simulink model "AutonomousDriving"  (R2018a)
settings: Solver=FixedStepAuto  StartTime=0.0  StopTime=inf  FixedStep=0.1  RelTol=1e-3
values from neighbouring files (symbols this model uses):
  init =     [init.mat]
undefined symbols (not defined in the file or in its folder): gray, Rec, SDTV
libraries: vrlib x7, visiontextngfix x4, visiontransforms x4, visiongeotforms x3, visionanalysis x3, visionstatistics x3, visionconversions x1
settings Model: Creator=al.hermann  LastModifiedBy=al.hermann

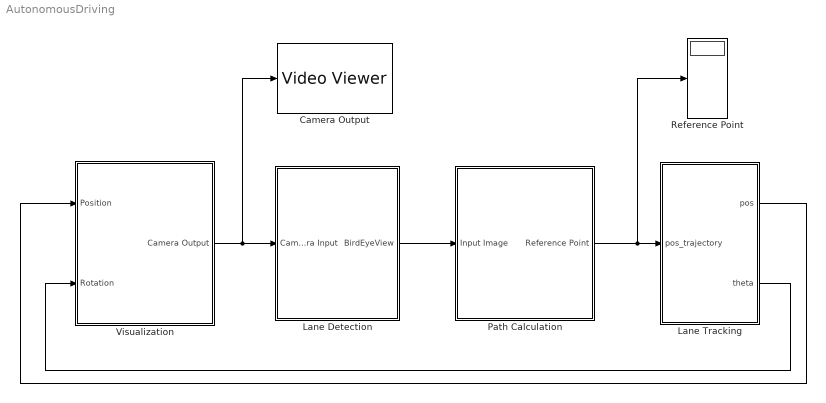
== system AutonomousDriving ==
  Camera Output : VideoViewer  colormapValue=gray(256)  FigPos=[1 481 575 361]
  Lane Detection : Subsystem
  Lane Tracking : Subsystem
  Path Calculation : Subsystem
  Reference Point : Display
  Visualization : Subsystem
  wires:
  Lane Detection/1(BirdEyeView) -> Path Calculation/1(Input Image)
  Lane Tracking/2(theta) -> Visualization/2(Rotation)
  Visualization/1(Camera Output) -> Lane Detection/1(Camera Input), Camera Output/1
  Lane Tracking/1(pos) -> Visualization/1(Position)
  Path Calculation/1("Reference Point ") -> Lane Tracking/1(pos_trajectory), Reference Point/1

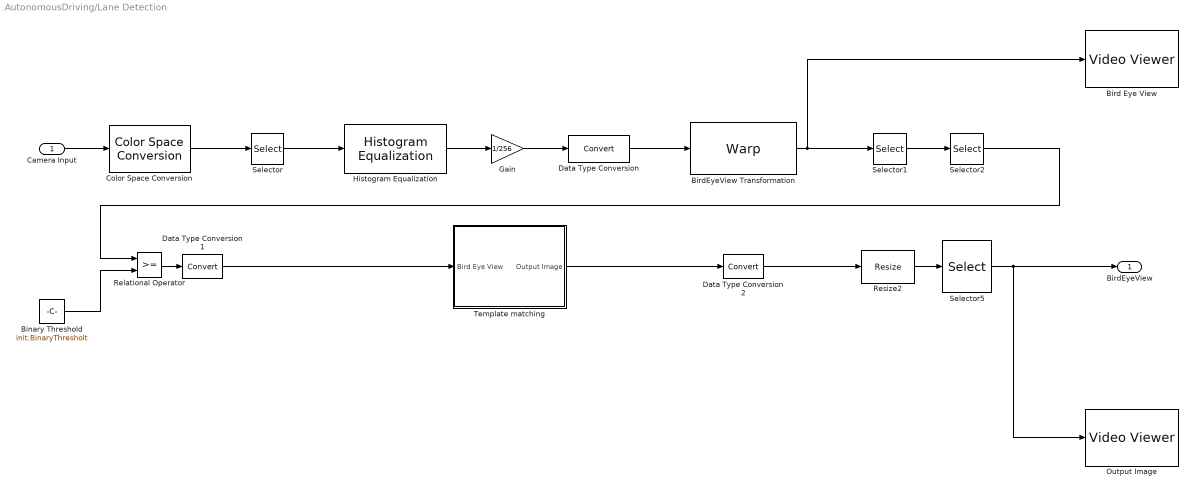
== system AutonomousDriving/Lane Detection ==
  Camera Input : Inport
  Binary Threshold : Constant  Value=init.BinaryThresholt
  Bird Eye View : VideoViewer  colormapValue=gray(256)  FigPos=[577 469 577 349]
  BirdEyeView Transformation : visiongeotforms/Warp  TransformMatrixSource=Custom  TransformMatrix=tf.T  InterpolationMethod=Bicubic  BackgroundFillValue=0  OutputImagePositionSource=Custom  OutputImagePosition=[-128, -128, 512, 512 ]  ROIInputPort=off  ROIValidityOutputPort=off  SimulateUsing=Interpreted execution
      settings: SourceProductName=Computer Vision System Toolbox  SourceProductBaseCode=VP
  Color Space Conversion : visionconversions/Color Space  Conversion  conversion=Obsolete  conversionActive=R'G'B' to intensity  wp_str=D65  rec=Rec. 601 (SDTV)  sys=1125/60/2:1  imagePorts=One multidimensional signal
      settings: SourceProductName=Computer Vision System Toolbox
  Data Type Conversion : DataTypeConversion
  Data Type Conversion1 : DataTypeConversion
  Data Type Conversion2 : DataTypeConversion
  Gain : Gain  Gain=1/256
  Histogram Equalization : visionanalysis/Histogram Equalization  specify=Uniform  numbins=256  src=Specify via dialog  hist=ones(1,64)
      settings: SourceProductName=Computer Vision System Toolbox  SourceProductBaseCode=VP
  Output Image : VideoViewer  colormapValue=gray(256)  FigPos=[519 965 488 384]
  Relational Operator : RelationalOperator  OutDataTypeStr=boolean  RndMeth=Simplest
  Resize2 : visiongeotforms/Resize  specify=Number of output rows and columns  rfactor=[500 100]  outCols=25  outRows=25  outRowsCols=init.ResizeImage  interp_method=Bilinear  antialias=on  useROI=off  roiFlag=off  prodOutputMode=Binary point scaling  prodOutputWordLength=32  prodOutputFracLength=10  roundingMode=Nearest  overflowMode=on
      settings: SourceProductName=Computer Vision System Toolbox  SourceProductBaseCode=VP
  Selector : Selector  NumberOfDimensions=2  InputPortWidth=3  IndexOptions=Starting index (dialog),Starting index (dialog)  Indices=100,50  OutputSizes=100,220
  Selector1 : Selector  NumberOfDimensions=2  InputPortWidth=3  IndexOptions=Starting index (dialog),Starting index (dialog)  Indices=244,1  OutputSizes=512-244,512
  Selector2 : Selector  NumberOfDimensions=2  InputPortWidth=3  IndexOptions=Starting index (dialog),Starting index (dialog)  Indices=1,1  OutputSizes=107,512
  Selector5 : Selector  NumberOfDimensions=2  InputPortWidth=3  IndexOptions=Starting index (dialog),Starting index (dialog)  Indices=25,50  OutputSizes=648-25,350
  Template matching : Subsystem
  BirdEyeView : Outport
  wires:
  Camera Input/1 -> Color Space Conversion/1
  Color Space Conversion/1 -> Selector/1
  Selector/1 -> Histogram Equalization/1
  Histogram Equalization/1 -> Gain/1
  Gain/1 -> Data Type Conversion/1
  Data Type Conversion/1 -> BirdEyeView Transformation/1
  Selector1/1 -> Selector2/1
  Relational Operator/1 -> Data Type Conversion1/1
  Binary Threshold/1 -> Relational Operator/2
  Data Type Conversion2/1 -> Resize2/1
  BirdEyeView Transformation/1 -> Selector1/1, Bird Eye View/1
  Selector2/1 -> Relational Operator/1
  Selector5/1 -> Output Image/1, BirdEyeView/1
  Resize2/1 -> Selector5/1
  Data Type Conversion1/1 -> Template matching/1(Bird Eye View)
  Template matching/1(Output Image) -> Data Type Conversion2/1

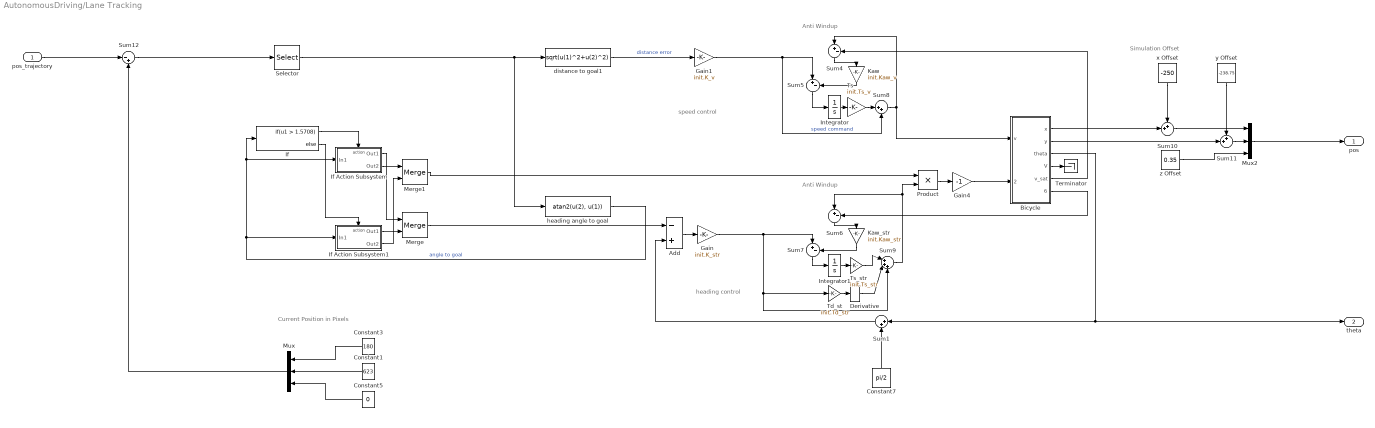
== system AutonomousDriving/Lane Tracking ==
  note: Simulation Offset
  note: Anti Windup
  note: Current Position in Pixels
  note: speed control
  note: heading control
  note: Anti Windup
  pos_trajectory : Inport
  Add : Sum  Inputs=-+
  Bicycle : Subsystem  AncestorBlock=roblocks/Vehicles/Bicycle  mask{vlim=init.v, accel=1, alim=120*pi/180, steer_rate=40*pi/180, L=2.812, x0=[0, 0, 0]}
      mask prompts: vlim "Velocity limit (m/s)"; accel "Acceleration limit (m/s2)"; alim "Steering angle limit (rad)"; steer_rate "Steering rate limit (rad/s)"; L "Wheel base"; x0 "Initial state (x, y, theta)"
      mask help: Kino-dynamic model of bicycle vehicle
      mask Help:
      | Kino-dynamic model of bicycle vehicle, also known as Ackermann vehicle
      | model.
      | 
      | <b>Parameters::</b>
      | 
      | Acceleration (1x1)   Vehicle acceleration limit [m/s2]
      | Velocity limit (1x1)  Vehicle speed limit [m/s]
      | Steering limits (1x1) Steering angle limit [rad]
      | Initial state (1x3) Initial state (x, y, theta)
      | Handbrake (1x1) Vehicle cannot move if non-zero
      | 
      | <b>Inputs::</b>
      | 
      | v (1x1) velocity demand [m/s]
      | gamma (1x1) steering angle [rad]
      | 
      | <b>Outputs::</b>
      | 
      | x (1x1) x-coordinate in world frame [m]
      | y (1x1) x-coordinate in world frame [m]
      | theta (1x1) heading angle in world frame [rad]
      | 
      | 
      | <b>Notes::</b>
      | 
      | - Steering limit is symmetric between -limit and +limit
      | - Same dynamic model as the Toolbox class Vehicle.
      mask Display:
      | port_label('input', 1, 'v')
      | port_label('input', 2, '\gamma', 'texmode', 'on')
      | port_label('output', 1, 'x')
      | port_label('output', 2, 'y')
      | port_label('output', 3, '\theta', 'texmode', 'on')
      | port_label('output', 4, 'v')
      | port_label('output', 5, 'v_{sat}', 'texmode', 'on')
      | port_label('output', 6, '\theta_{sat}', 'texmode', 'on')
  Constant1 : Constant  Value=623
  Constant3 : Constant  Value=180
  Constant5 : Constant  Value=0
  Constant7 : Constant  Value=pi/2
  Derivative : Derivative  CoefficientInTFapproximation=100
  Gain : Gain  Gain=init.K_str
  Gain1 : Gain  Gain=init.K_v
  Gain4 : Gain  Gain=-1
  If : If  IfExpression=u1 > 1.5708
  If Action Subsystem : Subsystem  TreatAsAtomicUnit=on
  If Action Subsystem1 : Subsystem  TreatAsAtomicUnit=on
  Integrator : Integrator
  Integrator1 : Integrator
  Kaw : Gain  Gain=init.Kaw_v
  Kaw_str : Gain  Gain=init.Kaw_str
  Merge : Merge
  Merge1 : Merge
  Mux : Mux  Inputs=3
  Mux2 : Mux  Inputs=3
  Product : Product
  Selector : Selector  InputPortWidth=3  IndexOptions=Index vector (dialog)  Indices=[1 2]  OutputSizes=1
  Sum1 : Sum  Inputs=|++
  Sum10 : Sum  Inputs=++|
  Sum11 : Sum  Inputs=++|
  Sum12 : Sum  Inputs=|-+
  Sum{4..7} (4 alike) : Sum  Inputs=|+-
  Sum8 : Sum  Inputs=|++
  Sum9 : Sum  Inputs=|+++
  Td_st : Gain  Gain=init.Td_str
  Terminator : Terminator
  Ts : Gain  Gain=init.Ts_v
  Ts_str : Gain  Gain=init.Ts_str
  distance to goal1 : Fcn  Expr=sqrt(u(1)^2+u(2)^2)
  heading angle to goal : Fcn  Expr=atan2(u(2), u(1))
  x Offset : Constant  Value=-250
  y Offset : Constant  Value=-238.75
  z Offset : Constant  Value=0.35
  pos : Outport
  theta : Outport  Port=2
  wires:
  pos_trajectory/1 -> Sum12/1
  distance to goal1/1 -> Gain1/1  "distance error"
  Bicycle/3(theta) -> Sum1/1, theta/1
  Sum12/1 -> Selector/1
  Selector/1 -> distance to goal1/1, heading angle to goal/1
  Mux/1 -> Sum12/2
  Constant1/1 -> Mux/2
  Constant3/1 -> Mux/1
  Constant7/1 -> Sum1/2
  Gain1/1 -> Sum8/2, Sum5/1  "speed command"
  Constant5/1 -> Mux/3
  Bicycle/1(x) -> Sum10/2
  Bicycle/2(y) -> Sum11/2
  If Action Subsystem/1(Out1) -> Merge/1
  If/1 -> If Action Subsystem/Action
  If/2 -> If Action Subsystem1/Action
  If Action Subsystem/2(Out2) -> Merge1/1
  If Action Subsystem1/1(Out1) -> Merge/2
  Bicycle/5("v_sat ") -> Sum4/2
  Sum4/1 -> Kaw/1
  Kaw/1 -> Sum5/2
  Sum5/1 -> Integrator/1
  Integrator/1 -> Ts/1
  Kaw_str/1 -> Sum7/2
  Sum7/1 -> Integrator1/1
  Sum6/1 -> Kaw_str/1
  Integrator1/1 -> Ts_str/1
  Ts/1 -> Sum8/1
  Bicycle/6("gamma_sat ") -> Sum6/2
  Gain/1 -> Sum9/3, Td_st/1, Sum7/1
  Ts_str/1 -> Sum9/1
  Derivative/1 -> Sum9/2
  Td_st/1 -> Derivative/1
  Sum8/1 -> Bicycle/1(v), Sum4/1
  x Offset/1 -> Sum10/1
  y Offset/1 -> Sum11/1
  Sum10/1 -> Mux2/1
  Sum11/1 -> Mux2/2
  z Offset/1 -> Mux2/3
  Mux2/1 -> pos/1
  Merge1/1 -> Product/1
  Product/1 -> Gain4/1
  If Action Subsystem1/2(Out2) -> Merge1/2
  Sum1/1 -> Add/2
  Add/1 -> Gain/1
  heading angle to goal/1 -> If Action Subsystem/1(In1), If/1, If Action Subsystem1/1(In1)  "angle to goal"
  Sum9/1 -> Sum6/1, Product/2
  Gain4/1 -> Bicycle/2(gamma)
  Merge/1 -> Add/1
  Bicycle/4(V) -> Terminator/1

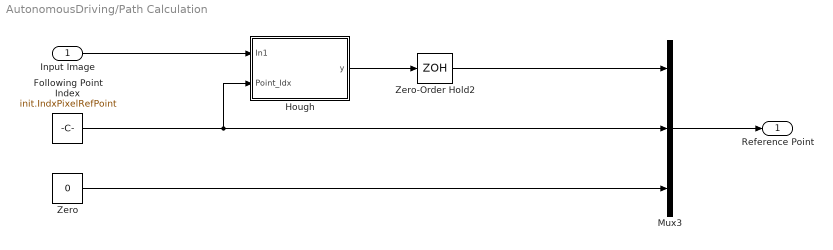
== system AutonomousDriving/Path Calculation ==
  Input Image : Inport
  Following Point Index : Constant  Value=init.IndxPixelRefPoint
  Hough : Subsystem
  Mux3 : Mux  Inputs=3
  Zero : Constant  Value=0
  Zero-Order Hold2 : ZeroOrderHold  SampleTime=0.2
  "Reference Point " : Outport
  wires:
  Input Image/1 -> Hough/1(In1)
  Hough/1(y) -> Zero-Order Hold2/1
  Zero-Order Hold2/1 -> Mux3/1
  Following Point Index/1 -> Hough/2(Point_Idx), Mux3/2
  Zero/1 -> Mux3/3
  Mux3/1 -> "Reference Point "/1

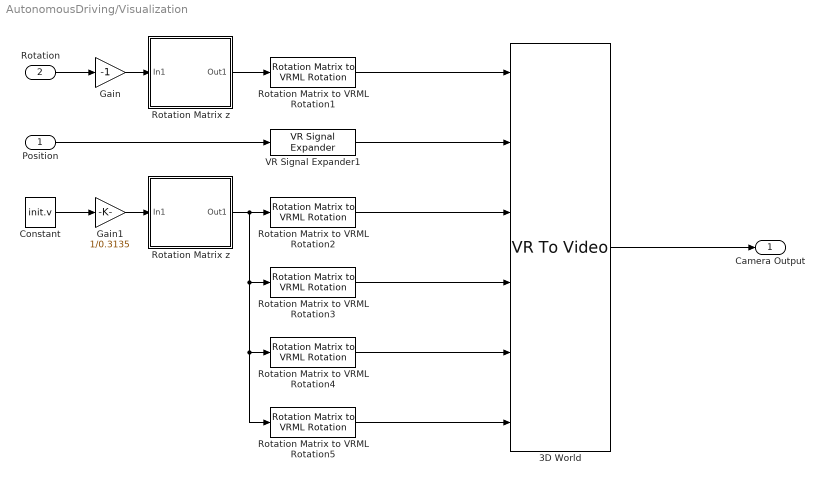
== system AutonomousDriving/Visualization ==
  Position : Inport
  Rotation : Inport  Port=2
  3D World : vrlib/VR To Video  InstantiateOnLoad=on  SampleTime=0.1  ViewEnable=on  RemoteChange=off  RemoteView=off  FieldsWritten=Car.rotation.4.1.1.double#Car.translation.3.1.1.double#RR_Rot.rotation.4.1.1.double#RL_Rot.rotation.4.1.1.double#FL_Rot.rotation.4.1.1.double#FR_Rot.rotation.4.1.1.double  WorldFileName=3DWorld.x3d  AutoView=off  VideoDimensions=[200 320]  AllowVariableSize=off  FigureProperties="{'Position', 'Name', 'Viewpoint', 'CameraBound', 'CameraDirection', 'CameraPosition', 'CameraUpVector', 'ZoomFactor', 'Antialiasing', 'Headlight', 'Lighting', 'NavPanel', 'Sound', 'StatusBar', 'Stereo3D', 'Stereo3DCameraOffset', 'Stereo3DHIT', 'ToolBar', 'Textures', 'Transparency', 'Triad', 'Wireframe', 'NavZones', 'NavMode', 'NavSpeed', 'CaptureFileFormat', 'CaptureFileName', 'Record2DCompressMethod', 'Record2DCompressQuality', 'Record2D', 'Record2DFileName', 'Record2DFPS'; [3.0000000000000000e+01   6.0000000000000000e+01   1.6000000000000000e+02   1.0000000000000000e+02], '', 'CAR', 'on', [0.0000000000000000e+00   0.0000000000000000e+00  -1.0000000000000000e+00], [0.0000000000000000e+00   0.0000000000000000e+00   0.0000000000000000e+00], [0.0000000000000000e+00   1.0000000000000000e+00   0.0000000000000000e+00], [1.0000000000000000e+00], 'on', 'on', 'on', 'none', 'on', 'off', 'off', [1.0000000149011612e-01], [0.0000000000000000e+00], 'off', 'on', 'on', 'none', 'off', 'off', 'examine', 'normal', 'tif', '%f_anim_%n.tif', 'auto', [7.5000000000000000e+01], 'off', '***video***', 'auto'}"
      settings: SourceProductName=Simulink 3D Animation  SourceProductBaseCode=VR
  Constant : Constant  Value=init.v
  Gain : Gain  Gain=-1
  Gain1 : Gain  Gain=1/0.3135
  Rotation Matrix to VRML Rotation{1..5} (5 alike) : vrlib/Utilities/Rotation Matrix to VRML Rotation  maxzero=1e-12
      settings: SourceProductName=Simulink 3D Animation  SourceProductBaseCode=VR
  Rotation Matrix z : Subsystem
  "Rotation Matrix z " : Subsystem
  VR Signal Expander1 : vrlib/VR Signal Expander  outwidth=3  outidx=[1 2 3]
      settings: SourceProductName=Simulink 3D Animation  SourceProductBaseCode=VR
  Camera Output : Outport
  wires:
  Rotation/1 -> Gain/1
  3D World/1 -> Camera Output/1
  Gain/1 -> Rotation Matrix z/1(In1)
  Position/1 -> VR Signal Expander1/1
  Rotation Matrix z/1(Out1) -> Rotation Matrix to VRML Rotation1/1
  Rotation Matrix to VRML Rotation1/1 -> 3D World/1
  VR Signal Expander1/1 -> 3D World/2
  Constant/1 -> Gain1/1
  Gain1/1 -> "Rotation Matrix z "/1(In1)
  "Rotation Matrix z "/1(Out1) -> Rotation Matrix to VRML Rotation3/1, Rotation Matrix to VRML Rotation5/1, Rotation Matrix to VRML Rotation4/1, Rotation Matrix to VRML Rotation2/1
  Rotation Matrix to VRML Rotation2/1 -> 3D World/3
  Rotation Matrix to VRML Rotation3/1 -> 3D World/4
  Rotation Matrix to VRML Rotation4/1 -> 3D World/5
  Rotation Matrix to VRML Rotation5/1 -> 3D World/6

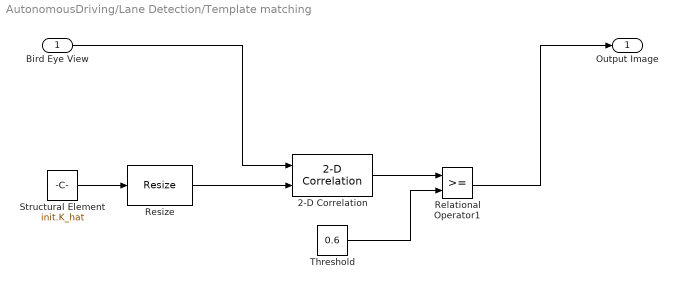
== system AutonomousDriving/Lane Detection/Template matching ==
  Bird Eye View : Inport
  2-D Correlation : visionstatistics/2-D Correlation  outSize=Full  normalize=on  roundingMode=Floor  overflowMode=off
      settings: SourceProductName=Computer Vision System Toolbox  SourceProductBaseCode=VP
  Relational Operator1 : RelationalOperator  OutDataTypeStr=boolean  RndMeth=Simplest
  Resize : visiongeotforms/Resize  specify=Number of output rows and columns  rfactor=[200 150]  outCols=25  outRows=25  outRowsCols=[6 6]  interp_method=Bilinear  antialias=on  useROI=off  roiFlag=off  prodOutputMode=Binary point scaling  prodOutputWordLength=32  prodOutputFracLength=10  roundingMode=Nearest  overflowMode=on
      settings: SourceProductName=Computer Vision System Toolbox  SourceProductBaseCode=VP
  Structural Element : Constant  Value=init.K_hat
  Threshold : Constant  Value=0.6
  Output Image : Outport
  wires:
  Bird Eye View/1 -> 2-D Correlation/1
  Relational Operator1/1 -> Output Image/1
  Threshold/1 -> Relational Operator1/2
  2-D Correlation/1 -> Relational Operator1/1
  Resize/1 -> 2-D Correlation/2
  Structural Element/1 -> Resize/1

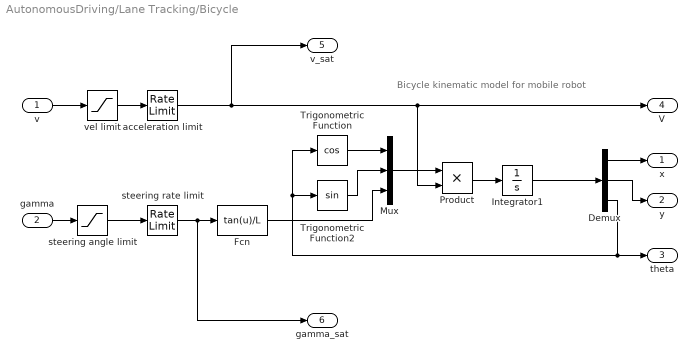
== system AutonomousDriving/Lane Tracking/Bicycle ==
  note: Bicycle kinematic model for mobile robot
  v : Inport
  gamma : Inport  Port=2
  Demux : Demux  Outputs=3
  Fcn : Fcn  Expr=tan(u)/L
  Integrator1 : Integrator  InitialCondition=x0
  Mux : Mux  Inputs=3
  Product : Product  RndMeth=Zero
  Trigonometric Function : Trigonometry  Operator=cos
  Trigonometric Function2 : Trigonometry
  acceleration limit : RateLimiter  RisingSlewLimit=accel  FallingSlewLimit=-accel  SampleTimeMode=inherited
  steering angle limit : Saturate  UpperLimit=alim  LowerLimit=-alim
  steering rate limit : RateLimiter  RisingSlewLimit=steer_rate  FallingSlewLimit=-steer_rate  SampleTimeMode=inherited
  vel limit : Saturate  UpperLimit=vlim  LowerLimit=-vlim
  x : Outport
  y : Outport  Port=2
  theta : Outport  Port=3
  V : Outport  Port=4
  "v_sat " : Outport  Port=5
  "gamma_sat " : Outport  Port=6
  wires:
  steering rate limit/1 -> "gamma_sat "/1, Fcn/1
  Product/1 -> Integrator1/1
  Integrator1/1 -> Demux/1
  Fcn/1 -> Mux/3
  Trigonometric Function/1 -> Mux/1
  acceleration limit/1 -> "v_sat "/1, V/1, Product/2
  Demux/3 -> Trigonometric Function/1, Trigonometric Function2/1, theta/1
  Demux/1 -> x/1
  Demux/2 -> y/1
  gamma/1 -> steering angle limit/1
  v/1 -> vel limit/1
  Mux/1 -> Product/1
  vel limit/1 -> acceleration limit/1
  Trigonometric Function2/1 -> Mux/2
  steering angle limit/1 -> steering rate limit/1

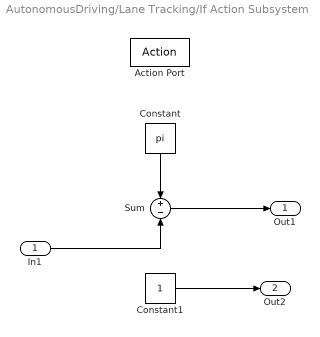
== system AutonomousDriving/Lane Tracking/If Action Subsystem ==
  In1 : Inport
  Action Port : ActionPort  ActionType=then
  Constant : Constant  Value=pi
  Constant1 : Constant
  Sum : Sum  Inputs=+-
  Out1 : Outport
  Out2 : Outport  Port=2
  wires:
  In1/1 -> Sum/2
  Sum/1 -> Out1/1
  Constant/1 -> Sum/1
  Constant1/1 -> Out2/1

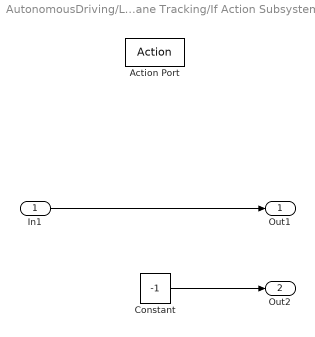
== system AutonomousDriving/Lane Tracking/If Action Subsystem1 ==
  In1 : Inport
  Action Port : ActionPort  ActionType=else
  Constant : Constant  Value=-1
  Out1 : Outport
  Out2 : Outport  Port=2
  wires:
  In1/1 -> Out1/1
  Constant/1 -> Out2/1

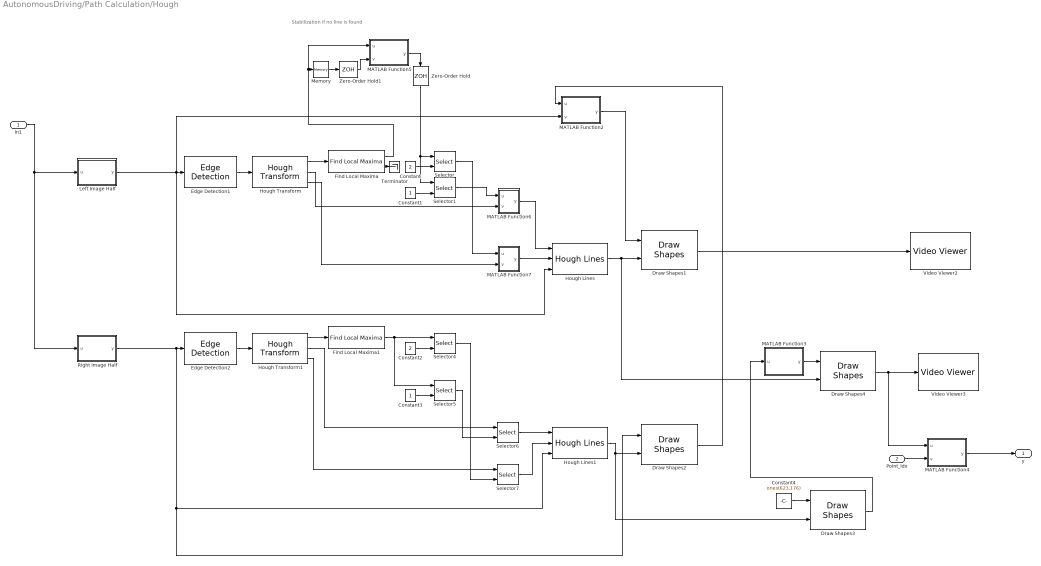
== system AutonomousDriving/Path Calculation/Hough ==
  note: Stabilization if no line is found
  In1 : Inport
  Point_Idx : Inport  Port=2
  Constant : Constant  Value=2
  Constant1 : Constant
  Constant2 : Constant  Value=2
  Constant3 : Constant
  Constant4 : Constant  Value=ones(623,176)
  Draw Shapes1 : visiontextngfix/Draw Shapes  shape=Lines  fill=off  lineWidth=5  fillClrSource=Specify via dialog  display=White  intensity=200  color=[200]  opacity=0.6  viewport=Entire image  antialiasing=off  inType=Obsolete  imagePorts=One multidimensional signal  prodOutputMode=Binary point scaling  prodOutputWordLength=32  prodOutputFracLength=14  memoryMode=Specify word length  memoryWordLength=16  memoryFracLength=14  roundingMode=Floor  overflowMode=off
      settings: SourceProductName=Computer Vision System Toolbox
  Draw Shapes2 : visiontextngfix/Draw Shapes  shape=Lines  fill=off  lineWidth=5  fillClrSource=Specify via dialog  display=White  intensity=200  color=[200 ]  opacity=0.6  viewport=Entire image  antialiasing=off  inType=Obsolete  imagePorts=One multidimensional signal  prodOutputMode=Binary point scaling  prodOutputWordLength=32  prodOutputFracLength=14  memoryMode=Specify word length  memoryWordLength=16  memoryFracLength=14  roundingMode=Floor  overflowMode=off
      settings: SourceProductName=Computer Vision System Toolbox
  Draw Shapes3 : visiontextngfix/Draw Shapes  shape=Lines  fill=off  lineWidth=5  fillClrSource=Specify via dialog  display=Black  intensity=200  color=[200 100 100]  opacity=0.6  viewport=Entire image  antialiasing=off  inType=Obsolete  imagePorts=One multidimensional signal  prodOutputMode=Binary point scaling  prodOutputWordLength=32  prodOutputFracLength=14  memoryMode=Specify word length  memoryWordLength=16  memoryFracLength=14  roundingMode=Floor  overflowMode=off
      settings: SourceProductName=Computer Vision System Toolbox
  Draw Shapes4 : visiontextngfix/Draw Shapes  shape=Lines  fill=off  lineWidth=5  fillClrSource=Specify via dialog  display=Black  intensity=200  color=[200 100 100]  opacity=0.6  viewport=Entire image  antialiasing=off  inType=Obsolete  imagePorts=One multidimensional signal  prodOutputMode=Binary point scaling  prodOutputWordLength=32  prodOutputFracLength=14  memoryMode=Specify word length  memoryWordLength=16  memoryFracLength=14  roundingMode=Floor  overflowMode=off
      settings: SourceProductName=Computer Vision System Toolbox
  Edge Detection1 : visionanalysis/Edge Detection  method=Canny  outputType=Binary image  userDefinedThreshold=off  thresholdSource=Input port  threshold=20  thresholdTuning=4  edgeThinning=off  threshold_canny=[0.25 0.60]  autoPercent=5  sigma=1  roundingMode=Floor  overflowMode=off  prodOutputMode=Binary point scaling  prodOutputWordLength=32  prodOutputFracLength=8  prodOutputSlope=2^-8  accumSlope=2^-8  outputSlope=2^-4
      settings: SourceProductName=Computer Vision System Toolbox  SourceProductBaseCode=VP
  Edge Detection2 : visionanalysis/Edge Detection  method=Canny  outputType=Binary image  userDefinedThreshold=off  thresholdSource=Input port  threshold=20  thresholdTuning=4  edgeThinning=off  threshold_canny=[0.25 0.60]  autoPercent=70  sigma=1  roundingMode=Floor  overflowMode=off  prodOutputMode=Binary point scaling  prodOutputWordLength=32  prodOutputFracLength=8  prodOutputSlope=2^-8  accumSlope=2^-8  outputSlope=2^-4
      settings: SourceProductName=Computer Vision System Toolbox  SourceProductBaseCode=VP
  Find Local Maxima : visionstatistics/Find Local Maxima  num_peaks=1  nhood_size=[3 3]  src_thresh=Obsolete9b  src_thresh_inuse=Specify via dialog  threshold=10  inputIsHough=on  dt_peak=uint32  isOutVarDim=off  dt_count=uint32
      settings: SourceProductName=Computer Vision System Toolbox  SourceProductBaseCode=VP
  Find Local Maxima1 : visionstatistics/Find Local Maxima  num_peaks=1  nhood_size=[3 3]  src_thresh=Obsolete9b  src_thresh_inuse=Specify via dialog  threshold=10  inputIsHough=on  dt_peak=uint32  isOutVarDim=on  dt_count=uint32
      settings: SourceProductName=Computer Vision System Toolbox  SourceProductBaseCode=VP
  Hough Lines : visiontransforms/Hough Lines  sineCompMethod=Trigonometric function  thetaRes=pi/180  firstCoeffMode=Specify word length  firstCoeffWordLength=16  firstCoeffFracLength=15  prodOutputMode=Binary point scaling  prodOutputWordLength=32  prodOutputFracLength=16  roundingMode=Nearest  overflowMode=on
      settings: SourceProductName=Computer Vision System Toolbox  SourceProductBaseCode=VP
  Hough Lines1 : visiontransforms/Hough Lines  sineCompMethod=Trigonometric function  thetaRes=pi/180  firstCoeffMode=Specify word length  firstCoeffWordLength=16  firstCoeffFracLength=15  prodOutputMode=Binary point scaling  prodOutputWordLength=32  prodOutputFracLength=16  roundingMode=Nearest  overflowMode=on
      settings: SourceProductName=Computer Vision System Toolbox  SourceProductBaseCode=VP
  Hough Transform : visiontransforms/Hough Transform  theta_res=pi/360  rho_res=1  out_theta_rho=on  outdtmode=double  firstCoeffMode=Binary point scaling  firstCoeffWordLength=16  firstCoeffFracLength=14  secondCoeffMode=Binary point scaling  secondCoeffWordLength=32  secondCoeffFracLength=16  outputMode=Binary point scaling  outputWordLength=16  outputFracLength=0  accumMode=Binary point scaling  accumWordLength=32  accumFracLength=20  prodOutputMode=Binary point scaling  prodOutputWordLength=32  prodOutputFracLength=20  memoryMode=Binary point scaling  memoryWordLength=32  memoryFracLength=16  roundingMode=Nearest  overflowMode=on
      settings: SourceProductName=Computer Vision System Toolbox  SourceProductBaseCode=VP
  Hough Transform1 : visiontransforms/Hough Transform  theta_res=pi/360  rho_res=1  out_theta_rho=on  outdtmode=double  firstCoeffMode=Binary point scaling  firstCoeffWordLength=16  firstCoeffFracLength=14  secondCoeffMode=Binary point scaling  secondCoeffWordLength=32  secondCoeffFracLength=16  outputMode=Binary point scaling  outputWordLength=16  outputFracLength=0  accumMode=Binary point scaling  accumWordLength=32  accumFracLength=20  prodOutputMode=Binary point scaling  prodOutputWordLength=32  prodOutputFracLength=20  memoryMode=Binary point scaling  memoryWordLength=32  memoryFracLength=16  roundingMode=Nearest  overflowMode=on
      settings: SourceProductName=Computer Vision System Toolbox  SourceProductBaseCode=VP
  Left Image Half : MATLAB Function  TreatAsAtomicUnit=on
  MATLAB Function2 : MATLAB Function  TreatAsAtomicUnit=on
  MATLAB Function3 : MATLAB Function  TreatAsAtomicUnit=on
  MATLAB Function4 : MATLAB Function  TreatAsAtomicUnit=on
  MATLAB Function5 : MATLAB Function  TreatAsAtomicUnit=on
  MATLAB Function6 : MATLAB Function  TreatAsAtomicUnit=on
  MATLAB Function7 : MATLAB Function  TreatAsAtomicUnit=on
  Memory : Memory
  Right Image Half : MATLAB Function  TreatAsAtomicUnit=on
  Selector : Selector  InputPortWidth=2  IndexOptions=Index vector (port)  Indices=1  OutputSizes=1
  Selector1 : Selector  InputPortWidth=2  IndexOptions=Index vector (port)  Indices=0  OutputSizes=1
  Selector4 : Selector  InputPortWidth=2  IndexOptions=Index vector (port)  Indices=1  OutputSizes=1
  Selector5 : Selector  InputPortWidth=2  IndexOptions=Index vector (port)  Indices=0  OutputSizes=1
  Selector6 : Selector  NumberOfDimensions=2  InputPortWidth=3  IndexOptions=Select all,Index vector (port)  Indices=[1 3],1  OutputSizes=1,1
  Selector7 : Selector  NumberOfDimensions=2  InputPortWidth=3  IndexOptions=Select all,Index vector (port)  Indices=[1 3],1  OutputSizes=1,1
  Terminator : Terminator
  Video Viewer2 : VideoViewer  colormapValue=gray(256)  FigPos=[1095 413 330 293]
  Video Viewer3 : VideoViewer  colormapValue=gray(256)  FigPos=[-7 981 517 409]
  Zero-Order Hold : ZeroOrderHold  SampleTime=0.2
  Zero-Order Hold1 : ZeroOrderHold  SampleTime=0.5
  y : Outport
  wires:
  Hough Transform/1 -> Find Local Maxima/1
  Selector7/1 -> Hough Lines1/2
  Draw Shapes1/1 -> Video Viewer2/1
  Constant1/1 -> Selector1/2
  Constant3/1 -> Selector5/2
  MATLAB Function7/1(y) -> Hough Lines/2
  Hough Lines1/1 -> Draw Shapes3/2, Draw Shapes2/2
  Constant2/1 -> Selector4/2
  Hough Transform1/2 -> Selector6/1
  Selector1/1 -> MATLAB Function6/1(u)
  In1/1 -> Left Image Half/1(u), Right Image Half/1(u)
  Selector5/1 -> Selector6/2
  Constant/1 -> Selector/2
  Hough Lines/1 -> Draw Shapes4/2, Draw Shapes1/2
  Hough Transform1/1 -> Find Local Maxima1/1
  Selector6/1 -> Hough Lines1/1
  Hough Transform1/3 -> Selector7/1
  Edge Detection1/1 -> Hough Transform/1
  Find Local Maxima1/1 -> Selector5/1, Selector4/1
  Draw Shapes2/1 -> MATLAB Function2/1(u)
  Edge Detection2/1 -> Hough Transform1/1
  Left Image Half/1(y) -> MATLAB Function2/2(v), Hough Lines/3, Edge Detection1/1
  Selector4/1 -> Selector7/2
  MATLAB Function6/1(y) -> Hough Lines/1
  Right Image Half/1(y) -> Draw Shapes2/1, Hough Lines1/3, Edge Detection2/1
  MATLAB Function2/1(y) -> Draw Shapes1/1
  Draw Shapes3/1 -> MATLAB Function3/1(u)
  MATLAB Function3/1(y) -> Draw Shapes4/1
  Draw Shapes4/1 -> MATLAB Function4/1(u), Video Viewer3/1
  Constant4/1 -> Draw Shapes3/1
  MATLAB Function4/1(y) -> y/1
  Point_Idx/1 -> MATLAB Function4/2(v)
  Find Local Maxima/1 -> MATLAB Function5/1(u), Memory/1
  Find Local Maxima/2 -> Terminator/1
  Hough Transform/2 -> MATLAB Function6/2(v)
  Memory/1 -> Zero-Order Hold1/1
  MATLAB Function5/1(y) -> Zero-Order Hold/1
  Hough Transform/3 -> MATLAB Function7/2(v)
  Selector/1 -> MATLAB Function7/1(u)
  Zero-Order Hold/1 -> Selector/1, Selector1/1
  Zero-Order Hold1/1 -> MATLAB Function5/2(v)

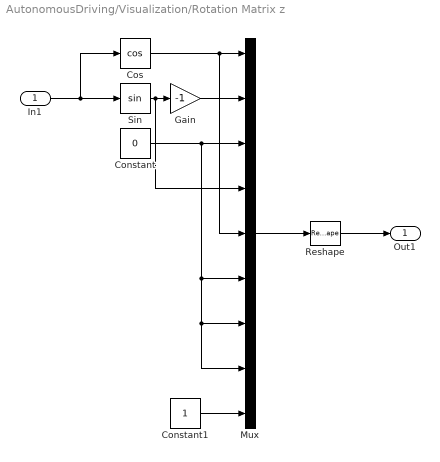
== system AutonomousDriving/Visualization/Rotation Matrix z ==
  In1 : Inport
  Constant : Constant  Value=0
  Constant1 : Constant
  Cos : Trigonometry  Operator=cos
  Gain : Gain  Gain=-1
  Mux : Mux  Inputs=9
  Reshape : Reshape  OutputDimensionality=Customize  OutputDimensions=[3, 3]
  Sin : Trigonometry
  Out1 : Outport
  wires:
  Reshape/1 -> Out1/1
  In1/1 -> Sin/1, Cos/1
  Mux/1 -> Reshape/1
  Cos/1 -> Mux/5, Mux/1
  Sin/1 -> Mux/4, Gain/1
  Constant/1 -> Mux/3, Mux/6, Mux/7, Mux/8
  Gain/1 -> Mux/2
  Constant1/1 -> Mux/9

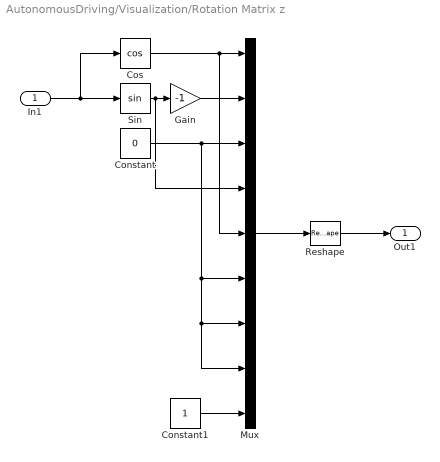
== system AutonomousDriving/Visualization/Rotation Matrix z  ==
  In1 : Inport
  Constant : Constant  Value=0
  Constant1 : Constant
  Cos : Trigonometry  Operator=cos
  Gain : Gain  Gain=-1
  Mux : Mux  Inputs=9
  Reshape : Reshape  OutputDimensionality=Customize  OutputDimensions=[3, 3]
  Sin : Trigonometry
  Out1 : Outport
  wires:
  Constant1/1 -> Mux/9
  Gain/1 -> Mux/2
  Constant/1 -> Mux/8, Mux/7, Mux/6, Mux/3
  Sin/1 -> Gain/1, Mux/4
  Cos/1 -> Mux/1, Mux/5
  Mux/1 -> Reshape/1
  In1/1 -> Cos/1, Sin/1
  Reshape/1 -> Out1/1

== matlab function AutonomousDriving/Path Calculation/Hough/Left Image Half ==
  data: u input; y output
function y = fcn(u)

y = u(1:end,1:size(u,2)/2,:);

== matlab function AutonomousDriving/Path Calculation/Hough/Right Image Half ==
  data: u input; y output
function y = fcn(u)

y = u(1:end,size(u,2)/2:end,:);

== matlab function AutonomousDriving/Path Calculation/Hough/MATLAB Function2 ==
  data: u input; y output; v input
function y = fcn(u, v)

y=ones(623,350);
y(:,1:350/2)=v;
y(:,350/2:end) = u;

== matlab function AutonomousDriving/Path Calculation/Hough/MATLAB Function3 ==
  data: u input; y output
function y = fcn(u)

y=ones(623,350);

y(:,350/2:end) = u;

== matlab function AutonomousDriving/Path Calculation/Hough/MATLAB Function4 ==
  data: u input; y output; v input
function y = fcn(u, v)

m=find(~u(v,:));

y = sum(m)/length(m);

== matlab function AutonomousDriving/Path Calculation/Hough/MATLAB Function5 ==
  data: u input; y output; v input
function y = fcn(u, v)

if u == 0
    
    y = v;
else 
    y = u;
end

== matlab function AutonomousDriving/Path Calculation/Hough/MATLAB Function6 ==
  data: u input; y output; v input
function y = fcn(u, v)

y = v(u+1);

== matlab function AutonomousDriving/Path Calculation/Hough/MATLAB Function7 ==
  data: u input; y output; v input
function y = fcn(u, v)

y = v(u+1);
